simulink model "CHUAN_LQG"  (R2017b)
settings: Solver=FixedStepAuto  StartTime=0.0  StopTime=30  FixedStep=0.01  RelTol=1e-3
values from neighbouring files (symbols this model uses):
  A = [0,                                                                                                                                                                                                                                                                1,                                                                                                                                            ...(+395 chars)    [CacFunctionTrongSimulink_LQR.m]    (also in QQQQ.m = [0 1 0 0; TINHGIATRIK.m = [0 1 0 0; TINHTHONGSOLQG.m = [0 1 0 0; Untitled3.m = [0,1,0,0)
  B = [                                                                                                                                                                                                                   0,                                                                                                                                                                                           ...(+27 chars)    [CacFunctionTrongSimulink_LQR.m]    (also in QQQQ.m = [ 0; TINHGIATRIK.m = [ 0; TINHTHONGSOLQG.m = [ 0; oke.m = [0 0; 0 0; 157.5798 157.5798; -75.9576 -75.9576; 0 0; -53.07)
  C = [1 0 0 0 ... (first row only)    [QQQQ.m]    (also in TINHGIATRIK.m; TINHTHONGSOLQG.m; pt_donghoc.m = [0,0,0,1]*inv([b,A*b,A^2*b,A^3*b])*(A-n1*eye(4))*(A-n2*eye(4)
  K = lqr(A,B,Q,R__)    [CacFunctionTrongSimulink_LQR.m]    (also in QQQQ.m = lqr(A,B,Q,R); TINHGIATRIK.m = lqr(A,B,Q,R); TINHTHONGSOLQG.m = lqr(A,B,Q,R))
  L = 0.08    [CacFunctionTrongSimulink_LQR.m]    (also in CacThongSoDongCo_LQR.m = 0.18; TINHTHONGSOLQG.m = lqe(A,G,C,Qn, Rn); pt_donghoc.m = 0.07)
libraries: simulink x2
settings Model: Creator=DELL  LastModifiedBy=DELL

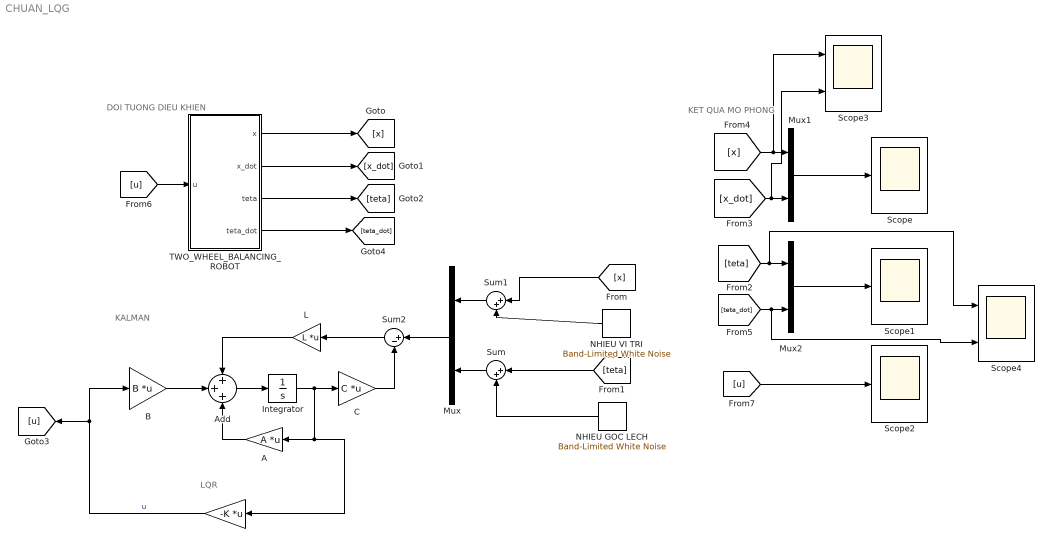
== system CHUAN_LQG ==
  note: DOI TUONG DIEU KHIEN
  note: KET QUA MO PHONG
  note: LQR
  note: KALMAN
  " " : Gain  Gain=-K  Multiplication=Matrix(K*u)
  A : Gain  Gain=A  Multiplication=Matrix(K*u)
  Add : Sum  Inputs=+++
  B : Gain  Gain=B  Multiplication=Matrix(K*u)
  C : Gain  Gain=C  Multiplication=Matrix(K*u)
  Integrator : Integrator
  L : Gain  Gain=L  Multiplication=Matrix(K*u)
  Mux : Mux  Inputs=2
  Mux1 : Mux  Inputs=2
  Mux2 : Mux  Inputs=2
  NHIEU GOC LECH : simulink/Sources/Band-Limited White Noise  Cov=[0.00000001]  Ts=0.01  seed=[23341]
  NHIEU VI TRI : simulink/Sources/Band-Limited White Noise  Cov=[0.000000001]  Ts=0.01  seed=[23341]
  Scope : Scope
  Scope1 : Scope
  Scope2 : Scope
  Scope3 : Scope  NumInputPorts=2
  Scope4 : Scope  NumInputPorts=2
  Sum : Sum  Inputs=|++
  Sum1 : Sum  Inputs=|++
  Sum2 : Sum  Inputs=|+-
  TWO_WHEEL_BALANCING_ROBOT : Subsystem
  wires:
  NHIEU VI TRI/1 -> Sum1/2
  C/1 -> Sum2/2
  " "/1 -> B/1, [u]  "u"
  TWO_WHEEL_BALANCING_ROBOT/2(x_dot) -> [x_dot]
  Sum2/1 -> L/1
  TWO_WHEEL_BALANCING_ROBOT/1(x) -> [x]
  Integrator/1 -> C/1, " "/1, A/1
  Mux/1 -> Sum2/1
  B/1 -> Add/2
  Add/1 -> Integrator/1
  L/1 -> Add/1
  A/1 -> Add/3
  Sum1/1 -> Mux/1
  TWO_WHEEL_BALANCING_ROBOT/3(teta) -> [teta]
  NHIEU GOC LECH/1 -> Sum/2
  Sum/1 -> Mux/2
  Mux1/1 -> Scope/1
  Mux2/1 -> Scope1/1
  [x] -> Sum1/1
  [teta] -> Sum/1
  [teta] -> Scope4/1, Mux2/1
  [x_dot] -> Scope3/2, Mux1/2
  [x] -> Scope3/1, Mux1/1
  TWO_WHEEL_BALANCING_ROBOT/4(teta_dot) -> [teta_dot]
  [teta_dot] -> Scope4/2, Mux2/2
  [u] -> TWO_WHEEL_BALANCING_ROBOT/1("u ")
  [u] -> Scope2/1

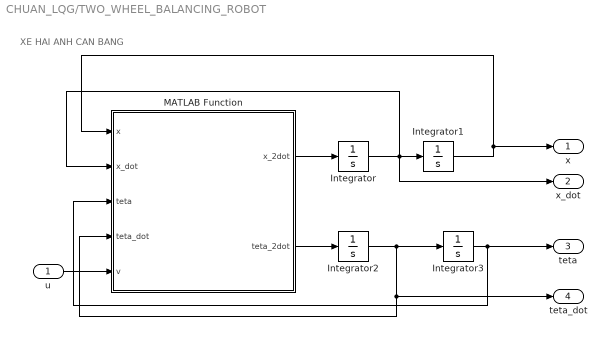
== system CHUAN_LQG/TWO_WHEEL_BALANCING_ROBOT ==
  note: XE HAI ANH CAN BANG
  "u " : Inport
  Integrator : Integrator
  Integrator1 : Integrator  InitialCondition=0.05
  Integrator2 : Integrator
  Integrator3 : Integrator  InitialCondition=0.05
  MATLAB Function : MATLAB Function  TreatAsAtomicUnit=on
  x : Outport
  x_dot : Outport  Port=2
  teta : Outport  Port=3
  teta_dot : Outport  Port=4
  wires:
  "u "/1 -> MATLAB Function/5(v)
  Integrator/1 -> x_dot/1, MATLAB Function/2(x_dot), Integrator1/1
  MATLAB Function/1(x_2dot) -> Integrator/1
  Integrator3/1 -> teta/1, MATLAB Function/3(teta)
  MATLAB Function/2(teta_2dot) -> Integrator2/1
  Integrator1/1 -> x/1, MATLAB Function/1(x)
  Integrator2/1 -> teta_dot/1, MATLAB Function/4(teta_dot), Integrator3/1

== matlab function CHUAN_LQG/TWO_WHEEL_BALANCING_ROBOT/MATLAB Function ==
  data: x input; x_2dot output; x_dot input; teta input; teta_dot input; v input; teta_2dot output
function [x_2dot,teta_2dot] = fcn(x,x_dot,teta,teta_dot,v)

g=9.81; %Gravity(m/s^2)
r=0.051; %Radius of wheel(m)
Mw=0.03; %Mass of wheel(kg)
Mp=1.13; %Mass of body(kg)
Iw=0.000039; %Inertia of the wheel(kg*m^2)
Ip=0.0041; %Inertia of the body(kg*m^2)
L=0.07; %Length to the body's center of mass(m)

%Motor's variables
Km=0.006123; %Motor torque constant(Nm/A)
Ke=0.006087; %Back EMF constant(Vs/rad)
R=3; %Nominal terminal resistance(Ohm)
a1=Mp*L/(Ip+Mp*L^2);
a2=Km*Ke/(R*r*(Ip+Mp*L^2));
a3=Km/(R*(Ip+Mp*L^2));
a4=Mp*g*L/(Ip+Mp*L^2);
b1=2*Km/(R*r*(2*Mw+2*(Iw/r^2)+Mp));
b2=2*Km*Ke/(R*r^2*(2*Mw+2*(Iw/r^2)+Mp));
b3=Mp*L/(2*Mw+2*(Iw/r^2)+Mp);
K=1.0e+03 *[-0.0316   -0.0361    1.6415    0.1272];
teta_2dot = -(a4*teta - 2*a3*v + 2*a2*x + a1*b1*v - a1*b2*x_dot)/(a1*b3 - 1);
x_2dot=-(b1*v - b2*x_dot + a4*b3*teta - 2*a3*b3*v + 2*a2*b3*x)/(a1*b3 - 1);
